simulink model "SCIM06"  (R2016a)
settings: Solver=FixedStepAuto  StartTime=0.0  StopTime=5  FixedStep=0.0001  RelTol=1e-3
values from neighbouring files (symbols this model uses):
  Lm = 0.1271    [motor4_workspace.mat]    (also in motor_wrapper.m = obj.Lm; scim_verifier.m = obj.motor.getLm(); setMotorParams.m; stationary_class.m = obj.Lm)
  Lr = 0.2744    [motor4_workspace.mat]    (also in motor_wrapper.m = obj.Lr; scim_verifier.m = obj.motor.getLr(); setMotorParams.m; stationary_class.m = obj.Lr)
  Ls = 0.2744    [motor4_workspace.mat]    (also in motor_wrapper.m = obj.Ls; scim_verifier.m = obj.motor.getLs(); setMotorParams.m; stationary.m = Ls/10)
  M_abc2ab0 = [0.666666666667  -0.333333333333  -0.333333333333; 0  0.57735026919  -0.57735026919; 0.333333333333  0.333333333333  0.333333333333]    [motor4_workspace.mat]    (also in setMotorParams.m = 2/3*[1, -0.5, -0.5; 0, sqrt(3)/2, -sqrt(3)/2;  0.5, 0.5, 0.5; workspaceSav.mat)
  R2 = 1.94147814274    [motor4_workspace.mat]    (also in setMotorParams.m; stationary_class.m = Rs+(Lm*Lm*Rr/Lr/Lr); torqueFinder.m; workspaceSav.mat = 7.05371900826)
  Rr = 1.009    [motor4_workspace.mat]    (also in motor_wrapper.m = obj.Rr; setMotorParams.m; stationary_class.m = obj.Rr; stationary_from_eq.m = obj.Rr)
  sig = (tox-fromx)/6    [gaussSpace.m]    (also in motor4_workspace.mat = 0.785452782217; setMotorParams.m = 0.785452782217; stationary_class.m = 1-Lm*Lm/Ls/Lr; torqueFinder.m = 0.785452782217)
settings Model: Creator=ebenera  LastModifiedBy=ebenera

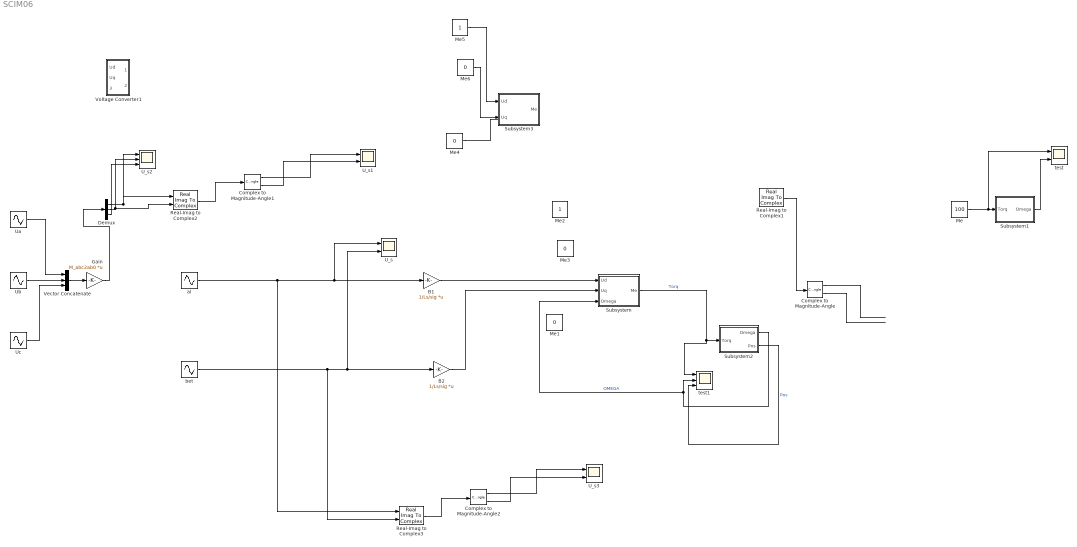
== system SCIM06 ==
  B1 : Gain  Gain=1/Ls/sig  Multiplication=Matrix(K*u)
  B2 : Gain  Gain=1/Ls/sig  Multiplication=Matrix(K*u)
  Complex to Magnitude-Angle : ComplexToMagnitudeAngle
  Complex to Magnitude-Angle1 : ComplexToMagnitudeAngle
  Complex to Magnitude-Angle2 : ComplexToMagnitudeAngle
  Demux : Demux  Outputs=3
  Gain : Gain  Gain=M_abc2ab0  Multiplication=Matrix(K*u)
  Me : Constant  Value=100
  Me{1,3..4,6} (4 alike) : Constant  Value=0
  Me2 : Constant
  Me5 : Constant
  Real-Imag to Complex1 : RealImagToComplex
  Real-Imag to Complex2 : RealImagToComplex
  Real-Imag to Complex3 : RealImagToComplex
  Subsystem : Subsystem
  Subsystem1 : Subsystem
  Subsystem2 : Subsystem
  Subsystem3 : Subsystem
  U_s : Scope  NumInputPorts=2
  U_s1 : Scope  NumInputPorts=2
  U_s2 : Scope  NumInputPorts=3
  U_s3 : Scope  NumInputPorts=2
  Ua : Sin  Amplitude=80  Frequency=314  SampleTime=0
  Ub : Sin  Amplitude=80  Frequency=314  Phase=-2*pi/3  SampleTime=0
  Uc : Sin  Amplitude=80  Frequency=314  Phase=2*pi/3  SampleTime=0
  Vector Concatenate : Concatenate  NumInputs=3
  Voltage Converter1 : Subsystem
  al : Sin  Amplitude=80  Frequency=314  Phase=1.57  SampleTime=0
  bet : Sin  Amplitude=80  Frequency=314  SampleTime=0
  test : Scope  NumInputPorts=2
  test1 : Scope  NumInputPorts=3
  wires:
  Subsystem2/2(Pos) -> test1/3  "Pos"
  Subsystem2/1(Omega) -> Subsystem/3(Omega), test1/2  "OMEGA"
  Me/1 -> test/1, Subsystem1/1("Torq ")
  Subsystem1/1(Omega) -> test/2
  Subsystem/1(Me) -> test1/1, Subsystem2/1("Torq ")  "Torq"
  Me4/1 -> ?
  Me5/1 -> Subsystem3/1(Ud)
  Me6/1 -> Subsystem3/2(Uq)
  B1/1 -> Subsystem/1(Ud)
  B2/1 -> Subsystem/2(Uq)
  al/1 -> Real-Imag to Complex3/1, U_s/1, B1/1
  bet/1 -> Real-Imag to Complex3/2, U_s/2, B2/1
  ? -> Real-Imag to Complex1/2  "I_sq"
  ? -> Real-Imag to Complex1/1  "I_sd"
  Real-Imag to Complex1/1 -> Complex to Magnitude-Angle/1
  Complex to Magnitude-Angle/1 -> ?
  Complex to Magnitude-Angle/2 -> ?
  Complex to Magnitude-Angle1/1 -> U_s1/1
  Complex to Magnitude-Angle1/2 -> U_s1/2
  Vector Concatenate/1 -> Gain/1
  Ua/1 -> Vector Concatenate/1
  Ub/1 -> Vector Concatenate/2
  Uc/1 -> Vector Concatenate/3
  Gain/1 -> Demux/1
  Demux/1 -> Real-Imag to Complex2/1, U_s2/1
  Demux/2 -> Real-Imag to Complex2/2, U_s2/2
  Demux/3 -> U_s2/3
  Real-Imag to Complex2/1 -> Complex to Magnitude-Angle1/1
  Complex to Magnitude-Angle2/1 -> U_s3/1
  Complex to Magnitude-Angle2/2 -> U_s3/2
  Real-Imag to Complex3/1 -> Complex to Magnitude-Angle2/1

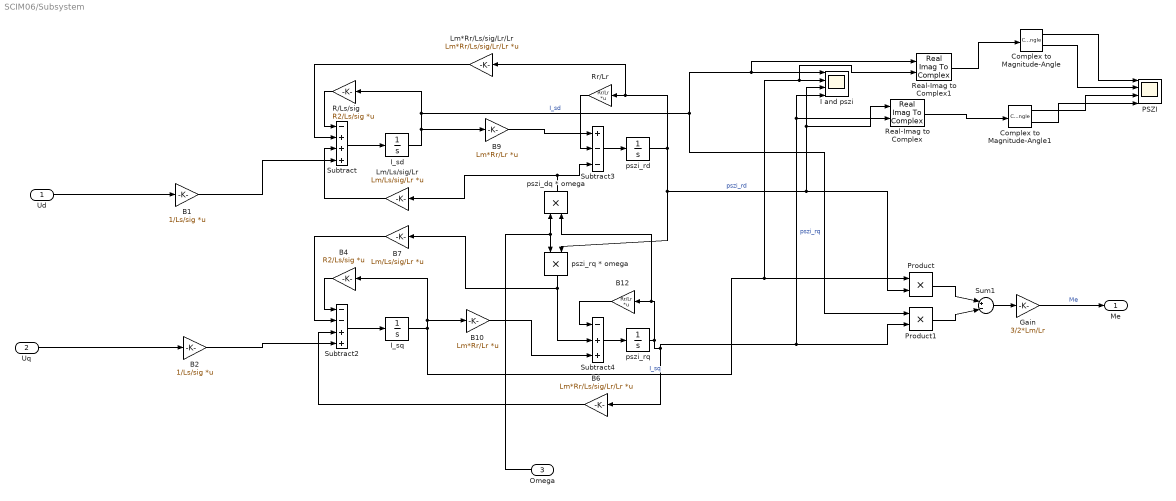
== system SCIM06/Subsystem ==
  Ud : Inport
  Uq : Inport  Port=2
  Omega : Inport  Port=3
  B1 : Gain  Gain=1/Ls/sig  Multiplication=Matrix(K*u)
  B10 : Gain  Gain=Lm*Rr/Lr  Multiplication=Matrix(K*u)
  B12 : Gain  Gain=Rr/Lr  Multiplication=Matrix(K*u)
  B2 : Gain  Gain=1/Ls/sig  Multiplication=Matrix(K*u)
  B4 : Gain  Gain=R2/Ls/sig  Multiplication=Matrix(K*u)
  B6 : Gain  Gain=Lm*Rr/Ls/sig/Lr/Lr  Multiplication=Matrix(K*u)
  B7 : Gain  Gain=Lm/Ls/sig/Lr  Multiplication=Matrix(K*u)
  B9 : Gain  Gain=Lm*Rr/Lr  Multiplication=Matrix(K*u)
  Complex to Magnitude-Angle : ComplexToMagnitudeAngle
  Complex to Magnitude-Angle1 : ComplexToMagnitudeAngle
  Gain : Gain  Gain=3/2*Lm/Lr
  I and pszi : Scope  NumInputPorts=4
  I_sd : Integrator
  I_sq : Integrator
  Lm*Rr/Ls/sig/Lr/Lr : Gain  Gain=Lm*Rr/Ls/sig/Lr/Lr  Multiplication=Matrix(K*u)
  Lm/Ls/sig/Lr : Gain  Gain=Lm/Ls/sig/Lr  Multiplication=Matrix(K*u)
  PSZI : Scope  NumInputPorts=4
  Product : Product
  Product1 : Product
  R/Ls/sig : Gain  Gain=R2/Ls/sig  Multiplication=Matrix(K*u)
  Real-Imag to Complex : RealImagToComplex
  Real-Imag to Complex1 : RealImagToComplex
  Rr/Lr : Gain  Gain=Rr/Lr  Multiplication=Matrix(K*u)
  Subtract : Sum  Inputs=-+++
  Subtract2 : Sum  Inputs=--++
  Subtract3 : Sum  Inputs=+--
  Subtract4 : Sum  Inputs=-++
  Sum1 : Sum  Inputs=|+-|
  pszi_dq * omega : Product
  pszi_rd : Integrator
  "pszi_rq " : Integrator
  pszi_rq * omega : Product
  Me : Outport
  wires:
  pszi_rq * omega/1 -> Subtract4/2, B7/1
  Subtract/1 -> I_sd/1
  B12/1 -> Subtract4/1
  Product1/1 -> Sum1/2
  Lm*Rr/Ls/sig/Lr/Lr/1 -> Subtract/2
  Product/1 -> Sum1/1
  I_sq/1 -> Real-Imag to Complex1/2, I and pszi/2, Product/1, B10/1, B4/1  "I_sq"
  I_sd/1 -> B9/1, Product1/1, Real-Imag to Complex1/1, I and pszi/1, R/Ls/sig/1  "I_sd"
  Sum1/1 -> Gain/1
  R/Ls/sig/1 -> Subtract/1
  B6/1 -> Subtract2/3
  B4/1 -> Subtract2/1
  pszi_dq * omega/1 -> Subtract3/3, Lm/Ls/sig/Lr/1
  Omega/1 -> pszi_rq * omega/1, pszi_dq * omega/1
  B9/1 -> Subtract3/1
  Rr/Lr/1 -> Subtract3/2
  pszi_rd/1 -> Real-Imag to Complex/1, I and pszi/3, Product/2, pszi_rq * omega/2, Lm*Rr/Ls/sig/Lr/Lr/1, Rr/Lr/1  "pszi_rd"
  Lm/Ls/sig/Lr/1 -> Subtract/3
  "pszi_rq "/1 -> pszi_dq * omega/2, B12/1, Real-Imag to Complex/2, I and pszi/4, Product1/2, B6/1  "pszi_rq"
  B7/1 -> Subtract2/2
  Gain/1 -> Me/1  "Me"
  B10/1 -> Subtract4/3
  Subtract4/1 -> "pszi_rq "/1
  Subtract2/1 -> I_sq/1
  Subtract3/1 -> pszi_rd/1
  Uq/1 -> B2/1
  Ud/1 -> B1/1
  B1/1 -> Subtract/4
  B2/1 -> Subtract2/4
  Real-Imag to Complex1/1 -> Complex to Magnitude-Angle/1
  Complex to Magnitude-Angle/1 -> PSZI/1
  Complex to Magnitude-Angle/2 -> PSZI/2
  Real-Imag to Complex/1 -> Complex to Magnitude-Angle1/1
  Complex to Magnitude-Angle1/1 -> PSZI/3
  Complex to Magnitude-Angle1/2 -> PSZI/4

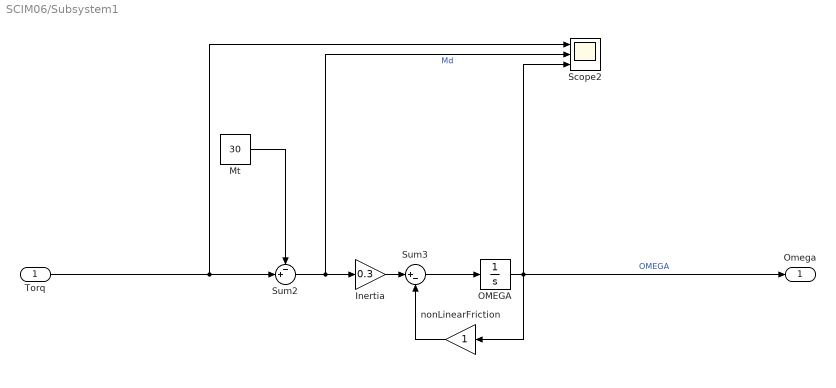
== system SCIM06/Subsystem1 ==
  "Torq " : Inport
  Inertia : Gain  Gain=0.3
  Mt : Constant  Value=30
  OMEGA : Integrator
  Scope2 : Scope  NumInputPorts=3
  Sum2 : Sum  Inputs=-+|
  Sum3 : Sum  Inputs=|+-
  nonLinearFriction : Gain
  Omega : Outport
  wires:
  "Torq "/1 -> Scope2/1, Sum2/2
  OMEGA/1 -> Scope2/3, Omega/1, nonLinearFriction/1  "OMEGA"
  Sum3/1 -> OMEGA/1
  Sum2/1 -> Inertia/1, Scope2/2  "Md"
  Mt/1 -> Sum2/1
  nonLinearFriction/1 -> Sum3/2
  Inertia/1 -> Sum3/1

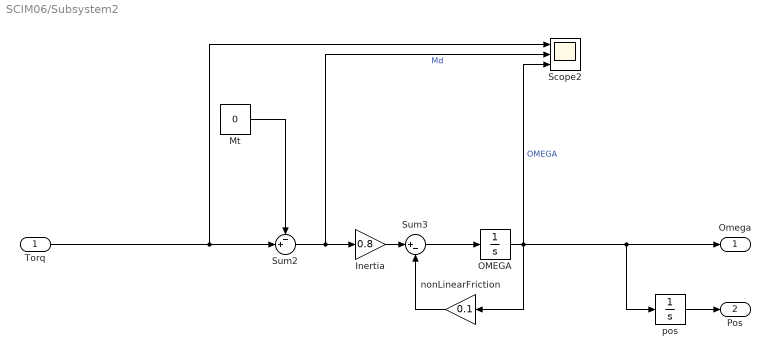
== system SCIM06/Subsystem2 ==
  "Torq " : Inport
  Inertia : Gain  Gain=0.8
  Mt : Constant  Value=0
  OMEGA : Integrator
  Scope2 : Scope  NumInputPorts=3
  Sum2 : Sum  Inputs=-+|
  Sum3 : Sum  Inputs=|+-
  nonLinearFriction : Gain  Gain=0.1
  pos : Integrator  WrapState=on
  Omega : Outport
  Pos : Outport  Port=2
  wires:
  "Torq "/1 -> Scope2/1, Sum2/2
  OMEGA/1 -> Scope2/3, pos/1, Omega/1, nonLinearFriction/1  "OMEGA"
  Sum3/1 -> OMEGA/1
  Sum2/1 -> Inertia/1, Scope2/2  "Md"
  Mt/1 -> Sum2/1
  nonLinearFriction/1 -> Sum3/2
  Inertia/1 -> Sum3/1
  pos/1 -> Pos/1

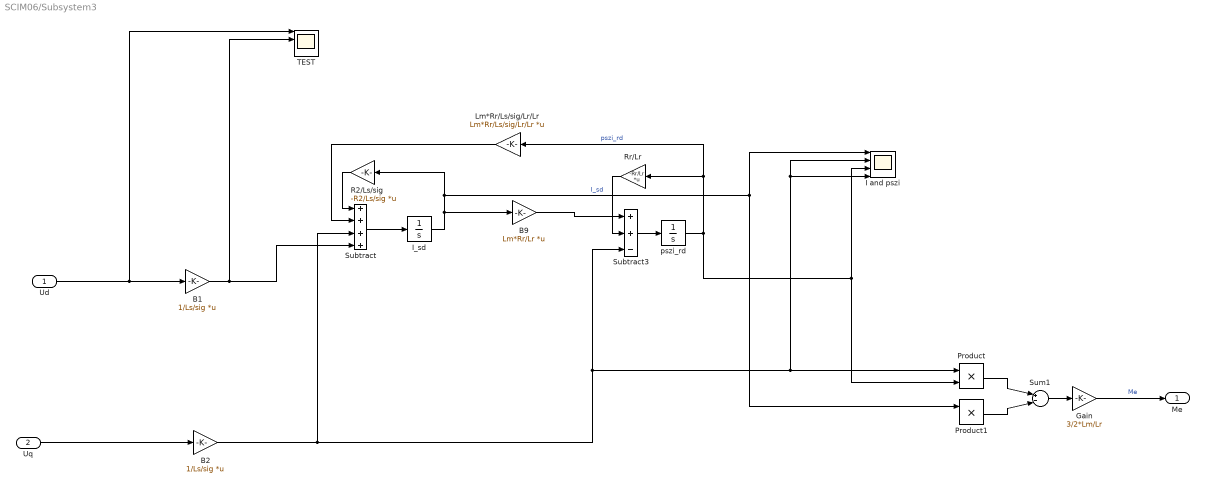
== system SCIM06/Subsystem3 ==
  Ud : Inport
  Uq : Inport  Port=2
  B1 : Gain  Gain=1/Ls/sig  Multiplication=Matrix(K*u)
  B2 : Gain  Gain=1/Ls/sig  Multiplication=Matrix(K*u)
  B9 : Gain  Gain=Lm*Rr/Lr  Multiplication=Matrix(K*u)
  Gain : Gain  Gain=3/2*Lm/Lr
  I and pszi : Scope  NumInputPorts=4
  I_sd : Integrator
  Lm*Rr/Ls/sig/Lr/Lr : Gain  Gain=Lm*Rr/Ls/sig/Lr/Lr  Multiplication=Matrix(K*u)
  Product : Product
  Product1 : Product
  R2/Ls/sig : Gain  Gain=-R2/Ls/sig  Multiplication=Matrix(K*u)
  Rr/Lr : Gain  Gain=-Rr/Lr  Multiplication=Matrix(K*u)
  Subtract : Sum  Inputs=++++
  Subtract3 : Sum  Inputs=++-
  Sum1 : Sum  Inputs=|+-|
  TEST : Scope  NumInputPorts=4
  pszi_rd : Integrator
  Me : Outport
  wires:
  Subtract/1 -> I_sd/1
  Product1/1 -> Sum1/2
  Lm*Rr/Ls/sig/Lr/Lr/1 -> Subtract/2
  Product/1 -> Sum1/1
  I_sd/1 -> B9/1, Product1/1, I and pszi/1, R2/Ls/sig/1  "I_sd"
  Sum1/1 -> Gain/1
  B9/1 -> Subtract3/1
  pszi_rd/1 -> I and pszi/3, Product/2, Lm*Rr/Ls/sig/Lr/Lr/1, Rr/Lr/1  "pszi_rd"
  Gain/1 -> Me/1  "Me"
  Subtract3/1 -> pszi_rd/1
  Uq/1 -> B2/1
  Ud/1 -> TEST/1, B1/1
  B1/1 -> TEST/2, Subtract/4
  B2/1 -> Subtract/3, Subtract3/3, Product/1, I and pszi/2, I and pszi/4
  Rr/Lr/1 -> Subtract3/2
  R2/Ls/sig/1 -> Subtract/1

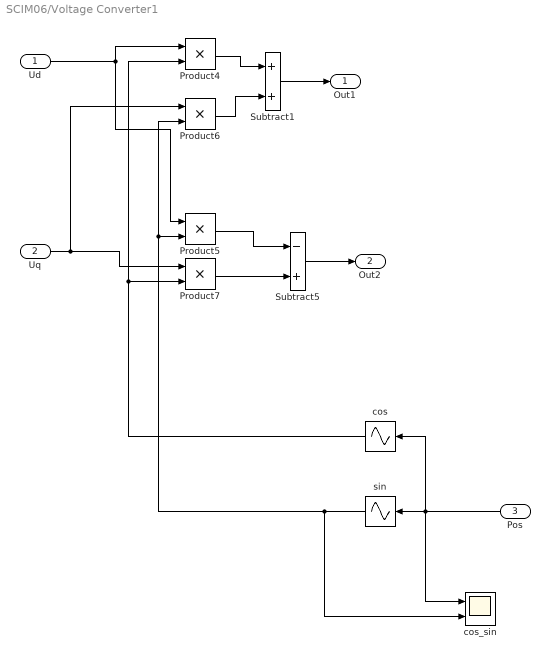
== system SCIM06/Voltage Converter1 ==
  Ud : Inport
  Uq : Inport  Port=2
  Pos : Inport  Port=3
  Product{4..7} (4 alike) : Product
  Subtract1 : Sum
  Subtract5 : Sum  Inputs=-+
  cos : Sin  TimeSource=Use external signal  Phase=+pi/2  SampleTime=0
  cos_sin : Scope  NumInputPorts=2
  sin : Sin  TimeSource=Use external signal  SampleTime=0
  Out1 : Outport
  Out2 : Outport  Port=2
  wires:
  cos/1 -> Product7/2, Product4/2
  Uq/1 -> Product6/1, Product7/1
  Ud/1 -> Product5/1, Product4/1
  Product4/1 -> Subtract1/1
  Product6/1 -> Subtract1/2
  Product5/1 -> Subtract5/1
  Product7/1 -> Subtract5/2
  Subtract5/1 -> Out2/1
  Subtract1/1 -> Out1/1
  sin/1 -> Product5/2, Product6/2, cos_sin/2
  Pos/1 -> cos_sin/1, sin/1, cos/1
